simulink model "ACDCMG_sim8"  (R2022a)
settings: Solver=FixedStepAuto  StartTime=0.0  StopTime=0.5  FixedStep=Ts  MaxStep=1e-2  RelTol=1e-3
InitFcn:
  | Set_parameters_R2018
values from neighbouring files (symbols this model uses):
  D_invs = 0.05    [Set_parameters_R2018.m]
  dis11 = 3    [Set_parameters_R2018.m]
  dis12 = 3    [Set_parameters_R2018.m]
  dis2 = 0.2    [Set_parameters_R2018.m]
  dis3 = 0.15    [Set_parameters_R2018.m]
  dis4 = 0.2    [Set_parameters_R2018.m]
  dis5 = 0.25    [Set_parameters_R2018.m]
  dis6 = 0.1    [Set_parameters_R2018.m]
  Fnom = 60    [Set_parameters_R2018.m]
  H_invs = 6    [Set_parameters_R2018.m]
  max_min = 1    [Set_parameters_R2018.m]
  P_Load_3 = S_Load_3* PF_Load_3    (= 7650)    [Set_parameters_R2018.m]
  P_nom_inv = 3e3    (= 3000)    [Set_parameters_R2018.m]
  Pnom_T1 = 1.5e6    (= 1500000)    [Set_parameters_R2018.m]
  Pnom_T2 = 1.5e6    (= 1500000)    [Set_parameters_R2018.m]
  Pnom_T3 = 4e6    (= 4000000)    [Set_parameters_R2018.m]
  Ql_Load_3 = S_Load_3 * sin(acos(PF_Load_3))    [Set_parameters_R2018.m]
  R_Load_9 = (Vnom_prim * 1.35)^2 / P_Load_9    (= 1084.6153125)    [Set_parameters_R2018.m]
  R_Load_DC = Vnom_DC^2/ P_Load_DC    (= 45)    [Set_parameters_R2018.m]
  Rl = 0.17    [Set_parameters_R2018.m]
  Rls = 0.013    [Set_parameters_R2018.m]
  Ts = Ts_Power    (= 6.94444444444e-06)    [Set_parameters_R2018.m]
  Ts_Control = 6*Ts_Power    (= 4.16666666667e-05)    [Set_parameters_R2018.m]
  Ts_Inv = 0.07    [Set_parameters_R2018.m]
  Ts_Power = 1/(24*Fnom)/100    (= 6.94444444444e-06)    [Set_parameters_R2018.m]
  Ts_PV = 0.05    [Set_parameters_R2018.m]
  V1_LL_T3 = 69e3    (= 69000)    [Set_parameters_R2018.m]
  Vmin_mppt = 100    [Set_parameters_R2018.m]
  Vnom_DC = 300    [Set_parameters_R2018.m]
  Vnom_Diesel = 2.4e3    (= 2400)    [Set_parameters_R2018.m]
  Vnom_prim = 13.8e3    (= 13800)    [Set_parameters_R2018.m]
  Vnom_sec = 220    [Set_parameters_R2018.m]
  Vnom_ter_AC_DC = 150    [Set_parameters_R2018.m]
  Xl = 0.3    [Set_parameters_R2018.m]
  Xls = 0.93e-3    (= 0.00093)    [Set_parameters_R2018.m]
undefined symbols (not defined in the file or in its folder): D1, dEgdT, Delta, DiscIntNeverNeededParam, EgRef, fn, gcbh, Ion, k1, Lithium, Rsh_array5pc, sps_rtmsupport, Tref_K, VnInv, VT_ref
libraries: spsCurrentMeasurementLib x40, spsRMSLib x29, spsSeriesRLCBranchLib x23, spsVoltageMeasurementLib x21, spsMeanLib x14, spsThreePhaseVIMeasurementLib x14, powerlib_extras x13, spsThreePhaseSeriesRLCBranchLib x12, spsPower3phInstantaneousLib x10, spsBreakerLib x8, spsControlledVoltageSourceLib x8, spsPowerLib x8
(part 2 of 12)

== system ACDCMG_sim8/SM_Grid_Simulation/Boost converter DC //DC 2 5 kHz - 300V  ==
  note: DC_PV Bus
  note: DC bus Bus
  note: 5 kHz - 300V
      | Boost Converter
  note: 10.5-kW Grid-Connected PV Array (Detailed Model)
  " " : Subsystem  mask(Boost Control - MPPT){fc=5000, T_MPPT=200e-6, Dinit=0.25}
      mask prompts: fc "PWM switching frequency (Hz)"; T_MPPT "Time window used by MPPT control (s)"; Dinit "Initial value of duty cycle"
      mask Display: image('Icons\FPGA.png');
  C1 : spsSeriesRLCBranchLib/Series RLC Branch  LConnTagsString=__new0  RConnTagsString=__new0  BranchType=C  Resistance=1.0  Inductance=1.0  SetiL0=off  InitialCurrent=0  Capacitance=1200e-6  Setx0=off  InitialVoltage=0  Measurements=None
  C3 : spsSeriesRLCBranchLib/Series RLC Branch  LConnTagsString=__new0  RConnTagsString=__new0  BranchType=C  Resistance=1.0  Inductance=1.0  SetiL0=off  InitialCurrent=0  Capacitance=100e-6  Setx0=off  InitialVoltage=0  Measurements=Branch voltage
  Current Measurement1 : spsCurrentMeasurementLib/Current Measurement  PhasorSimulation=off  OutputType=Complex  PSBequivalent=0
  Current Measurement2 : spsCurrentMeasurementLib/Current Measurement  PhasorSimulation=off  OutputType=Complex  PSBequivalent=0
  Diode1 : spsDiodeLib/Diode  Ron=1e-4  Lon=0  Vf=0  IC=0  UseSnubber=off  Rs=inf  Cs=inf  Measurements=off
  Display{2..4,6} (4 alike) : Display
  IGBT1 : spsIGBTLib/IGBT  Ron=0.001  Lon=0  Vf=0  Tf=0  Tt=0  IC=0  Rs=1e5  Cs=inf  Measurements=off
  L1 : spsSeriesRLCBranchLib/Series RLC Branch  LConnTagsString=__new0  RConnTagsString=__new0  BranchType=RL  Resistance=0.005  Inductance=9e-3  SetiL0=off  InitialCurrent=0  Capacitance=1e-6  Setx0=off  InitialVoltage=0  Measurements=None
  Mean : spsMeanLib/Mean  Freq=10  Vinit=0  Ts=0
  Mean1 : spsMeanLib/Mean  Freq=10  Vinit=0  Ts=0
  Product : Product
  Step : Step  Time=0  SampleTime=0
  "Vdc " : spsVoltageMeasurementLib/Voltage Measurement  Tag=PoWeRsYsTeMmEaSuReMeNt  PhasorSimulation=off  OutputType=Magnitude  PSBequivalent=0
  Vdc 1 : spsVoltageMeasurementLib/Voltage Measurement  Tag=PoWeRsYsTeMmEaSuReMeNt  PhasorSimulation=off  OutputType=Magnitude  PSBequivalent=0
  B + : PMIOPort  Side=Right
  + : PMIOPort  Port=2  Side=Left
  - : PMIOPort  Port=3  Side=Left
  B - : PMIOPort  Port=4  Side=Right
  tag scope: I_DC_bus_PV=global, V_DC_bus_PV=global, g_boost_PV=global
  wires:
  [I_PV] -> " "/2(I_PV)
  " "/1(Pulses) -> Product/2
  [V_PV] -> " "/1(V_PV)
  Step/1 -> Product/1
  Current Measurement2/1 -> Mean1/1
  Mean/1 -> Display6/1
  Current Measurement1/1 -> [I_DC_bus_PV], Mean/1
  "Vdc "/1 -> Display3/1, [V_DC_bus_PV]
  Product/1 -> [g_boost_PV]
  [g_boost_PV] -> IGBT1/1
  Vdc 1/1 -> Display4/1
  Mean1/1 -> Display2/1
  connections:
  Current Measurement2/RConn1 -- Vdc 1/LConn1 -- L1/LConn1 -- C3/LConn1
  C3/RConn1 -- -/RConn1 -- C1/RConn1 -- "Vdc "/LConn2 -- IGBT1/RConn1 -- B -/RConn1 -- Vdc 1/LConn2
  IGBT1/LConn1 -- Diode1/LConn1 -- L1/RConn1
  +/RConn1 -- Current Measurement1/RConn1
  C1/LConn1 -- Current Measurement1/LConn1 -- Diode1/RConn1 -- "Vdc "/LConn1
  B +/RConn1 -- Current Measurement2/LConn1

== system ACDCMG_sim8/SM_Grid_Simulation/Bus_1 ==
  Mux : Mux  Inputs=2
  "Power (3ph, Instantaneous)" : spsPower3phInstantaneousLib/Power (3ph, Instantaneous)
  Power Factor Block1 : Subsystem  mask(Power Factor Block){Freq=Fnom, Vinit=[0, 0], Iinit=[0, 0], Ts=0}
      mask prompts: Freq "Fundamental frequency (Hz):"; Vinit "Voltage initial input [ Mag, Phase (degrees) ]:"; Iinit "Current initial input [ Mag, Phase (degrees) ]:"; Ts "Sample time:"
      mask help:
      | Power Factor Block developed by Dr Rodney Tan
      | Version 1.01 (Aug 2016)
      |
      | Compute power factor and phase angle of AC circuit voltage-current pair at fundamental frequency.
      |
      | The computation is based on Power block and Complex number function block.
      |
      | For the first cycle of simulation, the outputs are held constant to the powers computed for the Voltage initial input and Current initial input parameters.
      mask Help:
      | <b>Fundamental Frequency (Hz)</b>
      | Specify the measurement fundamental frequency, in hertz, of the input signal.
      | 
      | <b>Voltage initial input [ Mag, Phase (degrees) ]</b>
      | Specify the voltage initial magnitude and phase to set a constant output for the first cycle of simulation.
      | 
      | <b>Current initial input [ Mag, Phase (degrees) ]</b>
      | Specify the current initial magnitude and phase to set a constant output for the first cycle of simulation.
      | 
      | <b>Sample Time</b>
      | Specify the sample time of the block, in seconds. Set to 0 to implement a continuous block.
      mask TypeOptions Freq: Power/Freq
      mask TypeOptions Vinit: Power/Vinit
      mask TypeOptions Iinit: Power/Iinit
      mask TypeOptions Ts: Power/Ts
  "Means_Bus1      " : Outport  VectorParamsAs1DForOutWhenUnconnected=off
  tag scope: Bus1_Iabc=global, Bus1_P=global, Bus1_Q=global, Bus1_Vabc=global
  wires:
  [IabcLL_Bus_1] -> "Power (3ph, Instantaneous)"/2, Power Factor Block1/2(Iabc), Mux/2  "Iabc"
  Mux/1 -> "Means_Bus1      "/1
  Power Factor Block1/2("Iabc y Iabc ") -> [Bus1_Iabc]
  Power Factor Block1/1("Vabc y Vabc ") -> [Bus1_Vabc]
  [VabcLL_Bus_1] -> Power Factor Block1/1(Vabc), "Power (3ph, Instantaneous)"/1, Mux/1  "Vabc"
  "Power (3ph, Instantaneous)"/1 -> [Bus1_P]
  "Power (3ph, Instantaneous)"/2 -> [Bus1_Q]

== system ACDCMG_sim8/SM_Grid_Simulation/Bus_14 1 ==
  " r1_ L13" : Constant  Value=Rl
  Active powers losses A : Display
      settings: Format=bank
  Active powers losses B : Display
      settings: Format=bank
  Active powers losses c : Display
      settings: Format=bank
  Math Function : Math  Operator=square  SignedPower=on
  Math Function1 : Math  Operator=square  SignedPower=on
  Math Function2 : Math  Operator=square  SignedPower=on
  Mux : Mux  Inputs=3
  Product : Product
  Product1 : Product
  Product2 : Product
  RMS1 : spsRMSLib/RMS  TrueRMS=on  Freq=60  RMSInit=0  Ts=0
  RMS2 : spsRMSLib/RMS  TrueRMS=on  Freq=60  RMSInit=0  Ts=0
  RMS3 : spsRMSLib/RMS  TrueRMS=on  Freq=60  RMSInit=0  Ts=0
  W_to_kW : Gain  Gain=1e-3
  W_to_kW1 : Gain  Gain=1e-3
  W_to_kW2 : Gain  Gain=1e-3
  tag scope: Bus_14_1_LineA_Ploss=global, Bus_14_1_LineB_Ploss=global, Bus_14_1_LineC_Ploss=global, Power_Losse_abc_L1=global
  wires:
  Math Function/1 -> Product/2
  [Ia_L1] -> RMS2/1
  Math Function1/1 -> Product1/2
  [Ib_L1] -> RMS1/1
  Math Function2/1 -> Product2/2
  " r1_ L13"/1 -> Product2/1, Product1/1, Product/1
  [Ic_L1] -> RMS3/1
  Product/1 -> W_to_kW/1
  Product2/1 -> W_to_kW2/1
  Product1/1 -> W_to_kW1/1
  RMS2/1 -> Math Function/1
  RMS1/1 -> Math Function1/1
  RMS3/1 -> Math Function2/1
  W_to_kW/1 -> [Bus_14_1_LineA_Ploss], Mux/1, Active powers losses A/1  "D_Pa_kW"
  W_to_kW1/1 -> [Bus_14_1_LineB_Ploss], Mux/2, Active powers losses B/1  "D_Pb_kW"
  W_to_kW2/1 -> Active powers losses c/1, [Bus_14_1_LineC_Ploss], Mux/3  "D_Pc_kW"
  Mux/1 -> [Power_Losse_abc_L1]

== system ACDCMG_sim8/SM_Grid_Simulation/Bus_14 2 ==
  " r1_ L13" : Constant  Value=Rls
  Active powers losses A : Display
      settings: Format=bank
  Active powers losses B : Display
      settings: Format=bank
  Active powers losses c : Display
      settings: Format=bank
  Math Function : Math  Operator=square  SignedPower=on
  Math Function1 : Math  Operator=square  SignedPower=on
  Math Function2 : Math  Operator=square  SignedPower=on
  Mux : Mux  Inputs=3
  Product : Product
  Product1 : Product
  Product2 : Product
  RMS1 : spsRMSLib/RMS  TrueRMS=on  Freq=60  RMSInit=0  Ts=0
  RMS2 : spsRMSLib/RMS  TrueRMS=on  Freq=60  RMSInit=0  Ts=0
  RMS3 : spsRMSLib/RMS  TrueRMS=on  Freq=60  RMSInit=0  Ts=0
  W_to_kW : Gain  Gain=1e-3
  W_to_kW1 : Gain  Gain=1e-3
  W_to_kW2 : Gain  Gain=1e-3
  tag scope: Bus_14_2_LineA_Ploss=global, Bus_14_2_LineB_Ploss=global, Bus_14_2_LineC_Ploss=global, Power_Losse_abc_L2=global
  wires:
  Math Function/1 -> Product/2
  [Ia_L2] -> RMS2/1
  Math Function1/1 -> Product1/2
  [Ib_L2] -> RMS1/1
  Math Function2/1 -> Product2/2
  " r1_ L13"/1 -> Product2/1, Product1/1, Product/1
  [Ic_L2] -> RMS3/1
  Product/1 -> W_to_kW/1
  Product2/1 -> W_to_kW2/1
  Product1/1 -> W_to_kW1/1
  RMS2/1 -> Math Function/1
  RMS1/1 -> Math Function1/1
  RMS3/1 -> Math Function2/1
  W_to_kW/1 -> [Bus_14_2_LineA_Ploss], Mux/1, Active powers losses A/1  "D_Pa_kW"
  W_to_kW1/1 -> [Bus_14_2_LineB_Ploss], Mux/2, Active powers losses B/1  "D_Pb_kW"
  W_to_kW2/1 -> Active powers losses c/1, [Bus_14_2_LineC_Ploss], Mux/3  "D_Pc_kW"
  Mux/1 -> [Power_Losse_abc_L2]

== system ACDCMG_sim8/SM_Grid_Simulation/Bus_14 3 ==
  " r1_ L13" : Constant  Value=Rl
  Active powers losses A : Display  Commented=on
      settings: Format=bank
  Active powers losses B : Display  Commented=on
      settings: Format=bank
  Active powers losses c : Display  Commented=on
      settings: Format=bank
  "Delta Pabc " : Scope  NumInputPorts=4
  Math Function : Math  Operator=square  SignedPower=on
  Math Function1 : Math  Operator=square  SignedPower=on
  Math Function2 : Math  Operator=square  SignedPower=on
  Mux : Mux  Inputs=3
  Product : Product
  Product1 : Product
  Product2 : Product
  RMS1 : spsRMSLib/RMS  TrueRMS=on  Freq=60  RMSInit=0  Ts=0
  RMS2 : spsRMSLib/RMS  TrueRMS=on  Freq=60  RMSInit=0  Ts=0
  RMS3 : spsRMSLib/RMS  TrueRMS=on  Freq=60  RMSInit=0  Ts=0
  W_to_kW : Gain  Gain=1e-3
  W_to_kW1 : Gain  Gain=1e-3
  W_to_kW2 : Gain  Gain=1e-3
  tag scope: Bus_14_3_LineA_Ploss=global, Bus_14_3_LineB_Ploss=global, Bus_14_3_LineC_Ploss=global, Power_Losse_abc_L3=global
  wires:
  Math Function/1 -> Product/2
  [Ia_L3] -> RMS2/1
  Math Function1/1 -> Product1/2
  [Ib_L3] -> RMS1/1
  Math Function2/1 -> Product2/2
  " r1_ L13"/1 -> Product2/1, Product1/1, Product/1
  [Ic_L3] -> RMS3/1
  Product/1 -> W_to_kW/1
  Product2/1 -> W_to_kW2/1
  Product1/1 -> W_to_kW1/1
  RMS2/1 -> Math Function/1
  RMS1/1 -> Math Function1/1
  RMS3/1 -> Math Function2/1
  W_to_kW/1 -> Mux/1, [Bus_14_3_LineA_Ploss], Active powers losses A/1  "D_Pa_kW"
  W_to_kW1/1 -> Mux/2, [Bus_14_3_LineB_Ploss], Active powers losses B/1  "D_Pb_kW"
  W_to_kW2/1 -> Active powers losses c/1, Mux/3, [Bus_14_3_LineC_Ploss]  "D_Pc_kW"
  Mux/1 -> [Power_Losse_abc_L3]

== system ACDCMG_sim8/SM_Grid_Simulation/Bus_14 4 ==
  " r1_ L13" : Constant  Value=Rls
  Active powers losses A : Display
      settings: Format=bank
  Active powers losses B : Display
      settings: Format=bank
  Active powers losses c : Display
      settings: Format=bank
  Math Function : Math  Operator=square  SignedPower=on
  Math Function1 : Math  Operator=square  SignedPower=on
  Math Function2 : Math  Operator=square  SignedPower=on
  Mux : Mux  Inputs=3
  Product : Product
  Product1 : Product
  Product2 : Product
  RMS1 : spsRMSLib/RMS  TrueRMS=on  Freq=60  RMSInit=0  Ts=0
  RMS2 : spsRMSLib/RMS  TrueRMS=on  Freq=60  RMSInit=0  Ts=0
  RMS3 : spsRMSLib/RMS  TrueRMS=on  Freq=60  RMSInit=0  Ts=0
  W_to_kW : Gain  Gain=1e-3
  W_to_kW1 : Gain  Gain=1e-3
  W_to_kW2 : Gain  Gain=1e-3
  tag scope: Bus_14_4_LineA_Ploss=global, Bus_14_4_LineB_Ploss=global, Bus_14_4_LineC_Ploss=global, Power_Losse_abc_L4=global
  wires:
  Math Function/1 -> Product/2
  [Ia_L4] -> RMS2/1
  Math Function1/1 -> Product1/2
  [Ib_L4] -> RMS1/1
  Math Function2/1 -> Product2/2
  " r1_ L13"/1 -> Product2/1, Product1/1, Product/1
  [Ic_L4] -> RMS3/1
  Product/1 -> W_to_kW/1
  Product2/1 -> W_to_kW2/1
  Product1/1 -> W_to_kW1/1
  RMS2/1 -> Math Function/1
  RMS1/1 -> Math Function1/1
  RMS3/1 -> Math Function2/1
  W_to_kW/1 -> Mux/1, [Bus_14_4_LineA_Ploss], Active powers losses A/1  "D_Pa_kW"
  W_to_kW1/1 -> Mux/2, [Bus_14_4_LineB_Ploss], Active powers losses B/1  "D_Pb_kW"
  W_to_kW2/1 -> Active powers losses c/1, [Bus_14_4_LineC_Ploss], Mux/3  "D_Pc_kW"
  Mux/1 -> [Power_Losse_abc_L4]

== system ACDCMG_sim8/SM_Grid_Simulation/Bus_14 5 ==
  " r1_ L13" : Constant  Value=Rls
  Active powers losses A : Display
      settings: Format=bank
  Active powers losses B : Display
      settings: Format=bank
  Active powers losses c : Display
      settings: Format=bank
  Math Function : Math  Operator=square  SignedPower=on
  Math Function1 : Math  Operator=square  SignedPower=on
  Math Function2 : Math  Operator=square  SignedPower=on
  Mux : Mux  Inputs=3
  Product : Product
  Product1 : Product
  Product2 : Product
  RMS1 : spsRMSLib/RMS  TrueRMS=on  Freq=60  RMSInit=0  Ts=0
  RMS2 : spsRMSLib/RMS  TrueRMS=on  Freq=60  RMSInit=0  Ts=0
  RMS3 : spsRMSLib/RMS  TrueRMS=on  Freq=60  RMSInit=0  Ts=0
  W_to_kW : Gain  Gain=1e-3
  W_to_kW1 : Gain  Gain=1e-3
  W_to_kW2 : Gain  Gain=1e-3
  tag scope: Bus_14_5_LineA_Ploss=global, Bus_14_5_LineB_Ploss=global, Bus_14_5_LineC_Ploss=global, Power_Losse_abc_L5=global
  wires:
  Math Function/1 -> Product/2
  [Ia_L5] -> RMS2/1
  Math Function1/1 -> Product1/2
  [Ib_L5] -> RMS1/1
  Math Function2/1 -> Product2/2
  " r1_ L13"/1 -> Product2/1, Product1/1, Product/1
  [Ic_L5] -> RMS3/1
  Product/1 -> W_to_kW/1
  Product2/1 -> W_to_kW2/1
  Product1/1 -> W_to_kW1/1
  RMS2/1 -> Math Function/1
  RMS1/1 -> Math Function1/1
  RMS3/1 -> Math Function2/1
  W_to_kW/1 -> [Bus_14_5_LineA_Ploss], Mux/1, Active powers losses A/1  "D_Pa_kW"
  W_to_kW1/1 -> [Bus_14_5_LineB_Ploss], Mux/2, Active powers losses B/1  "D_Pb_kW"
  W_to_kW2/1 -> Active powers losses c/1, [Bus_14_5_LineC_Ploss], Mux/3  "D_Pc_kW"
  Mux/1 -> [Power_Losse_abc_L5]

== system ACDCMG_sim8/SM_Grid_Simulation/Bus_14 6 ==
  " r1_ L13" : Constant  Value=Rls
  Active powers losses A : Display
      settings: Format=bank
  Active powers losses B : Display
      settings: Format=bank
  Active powers losses c : Display
      settings: Format=bank
  Math Function : Math  Operator=square  SignedPower=on
  Math Function1 : Math  Operator=square  SignedPower=on
  Math Function2 : Math  Operator=square  SignedPower=on
  Mux : Mux  Inputs=3
  Product : Product
  Product1 : Product
  Product2 : Product
  RMS1 : spsRMSLib/RMS  TrueRMS=on  Freq=60  RMSInit=0  Ts=0
  RMS2 : spsRMSLib/RMS  TrueRMS=on  Freq=60  RMSInit=0  Ts=0
  RMS3 : spsRMSLib/RMS  TrueRMS=on  Freq=60  RMSInit=0  Ts=0
  W_to_kW : Gain  Gain=1e-3
  W_to_kW1 : Gain  Gain=1e-3
  W_to_kW2 : Gain  Gain=1e-3
  tag scope: Bus_14_6_LineA_Ploss=global, Bus_14_6_LineB_Ploss=global, Bus_14_6_LineC_Ploss=global, Power_Losse_abc_L6=global
  wires:
  Math Function/1 -> Product/2
  [Ia_L6] -> RMS2/1
  Math Function1/1 -> Product1/2
  [Ib_L6] -> RMS1/1
  Math Function2/1 -> Product2/2
  " r1_ L13"/1 -> Product2/1, Product1/1, Product/1
  [Ic_L6] -> RMS3/1
  Product/1 -> W_to_kW/1
  Product2/1 -> W_to_kW2/1
  Product1/1 -> W_to_kW1/1
  RMS2/1 -> Math Function/1
  RMS1/1 -> Math Function1/1
  RMS3/1 -> Math Function2/1
  W_to_kW/1 -> [Bus_14_6_LineA_Ploss], Mux/1, Active powers losses A/1  "D_Pa_kW"
  W_to_kW1/1 -> [Bus_14_6_LineB_Ploss], Mux/2, Active powers losses B/1  "D_Pb_kW"
  W_to_kW2/1 -> Active powers losses c/1, [Bus_14_6_LineC_Ploss], Mux/3  "D_Pc_kW"
  Mux/1 -> [Power_Losse_abc_L6]

== system ACDCMG_sim8/SM_Grid_Simulation/Bus_14 7 ==
  " r1_ L13" : Constant  Value=Rls
  Active powers losses A : Display
      settings: Format=bank
  Active powers losses B : Display
      settings: Format=bank
  Active powers losses c : Display
      settings: Format=bank
  Math Function : Math  Operator=square  SignedPower=on
  Math Function1 : Math  Operator=square  SignedPower=on
  Math Function2 : Math  Operator=square  SignedPower=on
  Mux : Mux  Inputs=3
  Product : Product
  Product1 : Product
  Product2 : Product
  RMS1 : spsRMSLib/RMS  TrueRMS=on  Freq=60  RMSInit=0  Ts=0
  RMS2 : spsRMSLib/RMS  TrueRMS=on  Freq=60  RMSInit=0  Ts=0
  RMS3 : spsRMSLib/RMS  TrueRMS=on  Freq=60  RMSInit=0  Ts=0
  W_to_kW : Gain  Gain=1e-3
  W_to_kW1 : Gain  Gain=1e-3
  W_to_kW2 : Gain  Gain=1e-3
  tag scope: Bus_14_7_LineA_Ploss=global, Bus_14_7_LineB_Ploss=global, Bus_14_7_LineC_Ploss=global, Power_Losse_abc_L7=global
  wires:
  Math Function/1 -> Product/2
  [Ia_L7] -> RMS2/1
  Math Function1/1 -> Product1/2
  [Ib_L7] -> RMS1/1
  Math Function2/1 -> Product2/2
  " r1_ L13"/1 -> Product2/1, Product1/1, Product/1
  [Ic_L7] -> RMS3/1
  Product/1 -> W_to_kW/1
  Product2/1 -> W_to_kW2/1
  Product1/1 -> W_to_kW1/1
  RMS2/1 -> Math Function/1
  RMS1/1 -> Math Function1/1
  RMS3/1 -> Math Function2/1
  W_to_kW/1 -> [Bus_14_7_LineA_Ploss], Mux/1, Active powers losses A/1  "D_Pa_kW"
  W_to_kW1/1 -> [Bus_14_7_LineB_Ploss], Mux/2, Active powers losses B/1  "D_Pb_kW"
  W_to_kW2/1 -> Active powers losses c/1, [Bus_14_7_LineC_Ploss], Mux/3  "D_Pc_kW"
  Mux/1 -> [Power_Losse_abc_L7]

== system ACDCMG_sim8/SM_Grid_Simulation/Bus_2 ==
  "Power (3ph, Instantaneous)" : spsPower3phInstantaneousLib/Power (3ph, Instantaneous)
  Power Factor Block1 : Subsystem  mask(Power Factor Block){Freq=Fnom, Vinit=[0, 0], Iinit=[0, 0], Ts=0}
      mask prompts: Freq "Fundamental frequency (Hz):"; Vinit "Voltage initial input [ Mag, Phase (degrees) ]:"; Iinit "Current initial input [ Mag, Phase (degrees) ]:"; Ts "Sample time:"
      mask help:
      | Power Factor Block developed by Dr Rodney Tan
      | Version 1.01 (Aug 2016)
      |
      | Compute power factor and phase angle of AC circuit voltage-current pair at fundamental frequency.
      |
      | The computation is based on Power block and Complex number function block.
      |
      | For the first cycle of simulation, the outputs are held constant to the powers computed for the Voltage initial input and Current initial input parameters.
      mask Help:
      | <b>Fundamental Frequency (Hz)</b>
      | Specify the measurement fundamental frequency, in hertz, of the input signal.
      | 
      | <b>Voltage initial input [ Mag, Phase (degrees) ]</b>
      | Specify the voltage initial magnitude and phase to set a constant output for the first cycle of simulation.
      | 
      | <b>Current initial input [ Mag, Phase (degrees) ]</b>
      | Specify the current initial magnitude and phase to set a constant output for the first cycle of simulation.
      | 
      | <b>Sample Time</b>
      | Specify the sample time of the block, in seconds. Set to 0 to implement a continuous block.
      mask TypeOptions Freq: Power/Freq
      mask TypeOptions Vinit: Power/Vinit
      mask TypeOptions Iinit: Power/Iinit
      mask TypeOptions Ts: Power/Ts
  tag scope: Bus2_Iabc=global, Bus2_P=global, Bus2_Q=global, Bus2_Vabc=global
  wires:
  [IabcLL_Bus_2] -> "Power (3ph, Instantaneous)"/2, Power Factor Block1/2(Iabc)
  [VabcLL_Bus_2] -> "Power (3ph, Instantaneous)"/1, Power Factor Block1/1(Vabc)  "Vabc"
  "Power (3ph, Instantaneous)"/1 -> [Bus2_P]
  "Power (3ph, Instantaneous)"/2 -> [Bus2_Q]
  Power Factor Block1/1("Vabc y Vabc ") -> [Bus2_Vabc]
  Power Factor Block1/2("Iabc y Iabc ") -> [Bus2_Iabc]

== system ACDCMG_sim8/SM_Grid_Simulation/Bus_3 ==
  "Power (3ph, Instantaneous)" : spsPower3phInstantaneousLib/Power (3ph, Instantaneous)
  Power Factor Block1 : Subsystem  mask(Power Factor Block){Freq=Fnom, Vinit=[0, 0], Iinit=[0, 0], Ts=0}
      mask prompts: Freq "Fundamental frequency (Hz):"; Vinit "Voltage initial input [ Mag, Phase (degrees) ]:"; Iinit "Current initial input [ Mag, Phase (degrees) ]:"; Ts "Sample time:"
      mask help:
      | Power Factor Block developed by Dr Rodney Tan
      | Version 1.01 (Aug 2016)
      |
      | Compute power factor and phase angle of AC circuit voltage-current pair at fundamental frequency.
      |
      | The computation is based on Power block and Complex number function block.
      |
      | For the first cycle of simulation, the outputs are held constant to the powers computed for the Voltage initial input and Current initial input parameters.
      mask Help:
      | <b>Fundamental Frequency (Hz)</b>
      | Specify the measurement fundamental frequency, in hertz, of the input signal.
      | 
      | <b>Voltage initial input [ Mag, Phase (degrees) ]</b>
      | Specify the voltage initial magnitude and phase to set a constant output for the first cycle of simulation.
      | 
      | <b>Current initial input [ Mag, Phase (degrees) ]</b>
      | Specify the current initial magnitude and phase to set a constant output for the first cycle of simulation.
      | 
      | <b>Sample Time</b>
      | Specify the sample time of the block, in seconds. Set to 0 to implement a continuous block.
      mask TypeOptions Freq: Power/Freq
      mask TypeOptions Vinit: Power/Vinit
      mask TypeOptions Iinit: Power/Iinit
      mask TypeOptions Ts: Power/Ts
  tag scope: Bus3_Iabc=global, Bus3_P=global, Bus3_Q=global, Bus3_Vabc=global
  wires:
  [IabcLL_Bus_3] -> "Power (3ph, Instantaneous)"/2, Power Factor Block1/2(Iabc)
  [VabcLL_Bus_3] -> "Power (3ph, Instantaneous)"/1, Power Factor Block1/1(Vabc)  "Signal Vabc"
  "Power (3ph, Instantaneous)"/1 -> [Bus3_P]
  "Power (3ph, Instantaneous)"/2 -> [Bus3_Q]
  Power Factor Block1/1(Vabc y Vabc) -> [Bus3_Vabc]
  Power Factor Block1/2("Iabc y Iabc ") -> [Bus3_Iabc]

== system ACDCMG_sim8/SM_Grid_Simulation/Bus_4 ==
  "Power (3ph, Instantaneous)" : spsPower3phInstantaneousLib/Power (3ph, Instantaneous)
  Power Factor Block1 : Subsystem  mask(Power Factor Block){Freq=Fnom, Vinit=[0, 0], Iinit=[0, 0], Ts=0}
      mask prompts: Freq "Fundamental frequency (Hz):"; Vinit "Voltage initial input [ Mag, Phase (degrees) ]:"; Iinit "Current initial input [ Mag, Phase (degrees) ]:"; Ts "Sample time:"
      mask help:
      | Power Factor Block developed by Dr Rodney Tan
      | Version 1.01 (Aug 2016)
      |
      | Compute power factor and phase angle of AC circuit voltage-current pair at fundamental frequency.
      |
      | The computation is based on Power block and Complex number function block.
      |
      | For the first cycle of simulation, the outputs are held constant to the powers computed for the Voltage initial input and Current initial input parameters.
      mask Help:
      | <b>Fundamental Frequency (Hz)</b>
      | Specify the measurement fundamental frequency, in hertz, of the input signal.
      | 
      | <b>Voltage initial input [ Mag, Phase (degrees) ]</b>
      | Specify the voltage initial magnitude and phase to set a constant output for the first cycle of simulation.
      | 
      | <b>Current initial input [ Mag, Phase (degrees) ]</b>
      | Specify the current initial magnitude and phase to set a constant output for the first cycle of simulation.
      | 
      | <b>Sample Time</b>
      | Specify the sample time of the block, in seconds. Set to 0 to implement a continuous block.
      mask TypeOptions Freq: Power/Freq
      mask TypeOptions Vinit: Power/Vinit
      mask TypeOptions Iinit: Power/Iinit
      mask TypeOptions Ts: Power/Ts
  tag scope: Bus4_Iabc=global, Bus4_P=global, Bus4_Q=global, Bus4_Vabc=global
  wires:
  [IabcLL_Bus_4] -> "Power (3ph, Instantaneous)"/2, Power Factor Block1/2(Iabc)
  Power Factor Block1/2("Iabc y Iabc ") -> [Bus4_Iabc]
  Power Factor Block1/1(Vabc y Vabc) -> [Bus4_Vabc]
  [VabcLL_Bus_4] -> "Power (3ph, Instantaneous)"/1, Power Factor Block1/1(Vabc)  "Signal Vabc"
  "Power (3ph, Instantaneous)"/1 -> [Bus4_P]
  "Power (3ph, Instantaneous)"/2 -> [Bus4_Q]

== system ACDCMG_sim8/SM_Grid_Simulation/Bus_5 ==
  "Power (3ph, Instantaneous)" : spsPower3phInstantaneousLib/Power (3ph, Instantaneous)
  Power Factor Block1 : Subsystem  mask(Power Factor Block){Freq=Fnom, Vinit=[0, 0], Iinit=[0, 0], Ts=0}
      mask prompts: Freq "Fundamental frequency (Hz):"; Vinit "Voltage initial input [ Mag, Phase (degrees) ]:"; Iinit "Current initial input [ Mag, Phase (degrees) ]:"; Ts "Sample time:"
      mask help:
      | Power Factor Block developed by Dr Rodney Tan
      | Version 1.01 (Aug 2016)
      |
      | Compute power factor and phase angle of AC circuit voltage-current pair at fundamental frequency.
      |
      | The computation is based on Power block and Complex number function block.
      |
      | For the first cycle of simulation, the outputs are held constant to the powers computed for the Voltage initial input and Current initial input parameters.
      mask Help:
      | <b>Fundamental Frequency (Hz)</b>
      | Specify the measurement fundamental frequency, in hertz, of the input signal.
      | 
      | <b>Voltage initial input [ Mag, Phase (degrees) ]</b>
      | Specify the voltage initial magnitude and phase to set a constant output for the first cycle of simulation.
      | 
      | <b>Current initial input [ Mag, Phase (degrees) ]</b>
      | Specify the current initial magnitude and phase to set a constant output for the first cycle of simulation.
      | 
      | <b>Sample Time</b>
      | Specify the sample time of the block, in seconds. Set to 0 to implement a continuous block.
      mask TypeOptions Freq: Power/Freq
      mask TypeOptions Vinit: Power/Vinit
      mask TypeOptions Iinit: Power/Iinit
      mask TypeOptions Ts: Power/Ts
  tag scope: Bus5_Iabc=global, Bus5_P=global, Bus5_Q=global, Bus5_Vabc=global
  wires:
  [IabcLL_Bus_5] -> Power Factor Block1/2(Iabc), "Power (3ph, Instantaneous)"/2
  Power Factor Block1/2("Iabc y Iabc ") -> [Bus5_Iabc]
  Power Factor Block1/1(Vabc y Vabc) -> [Bus5_Vabc]
  [VabcLL_Bus_5] -> "Power (3ph, Instantaneous)"/1, Power Factor Block1/1(Vabc)  "Signal Vabc"
  "Power (3ph, Instantaneous)"/1 -> [Bus5_P]
  "Power (3ph, Instantaneous)"/2 -> [Bus5_Q]

== system ACDCMG_sim8/SM_Grid_Simulation/Bus_6 ==
  "Power (3ph, Instantaneous)" : spsPower3phInstantaneousLib/Power (3ph, Instantaneous)
  Power Factor Block1 : Subsystem  mask(Power Factor Block){Freq=Fnom, Vinit=[0, 0], Iinit=[0, 0], Ts=0}
      mask prompts: Freq "Fundamental frequency (Hz):"; Vinit "Voltage initial input [ Mag, Phase (degrees) ]:"; Iinit "Current initial input [ Mag, Phase (degrees) ]:"; Ts "Sample time:"
      mask help:
      | Power Factor Block developed by Dr Rodney Tan
      | Version 1.01 (Aug 2016)
      |
      | Compute power factor and phase angle of AC circuit voltage-current pair at fundamental frequency.
      |
      | The computation is based on Power block and Complex number function block.
      |
      | For the first cycle of simulation, the outputs are held constant to the powers computed for the Voltage initial input and Current initial input parameters.
      mask Help:
      | <b>Fundamental Frequency (Hz)</b>
      | Specify the measurement fundamental frequency, in hertz, of the input signal.
      | 
      | <b>Voltage initial input [ Mag, Phase (degrees) ]</b>
      | Specify the voltage initial magnitude and phase to set a constant output for the first cycle of simulation.
      | 
      | <b>Current initial input [ Mag, Phase (degrees) ]</b>
      | Specify the current initial magnitude and phase to set a constant output for the first cycle of simulation.
      | 
      | <b>Sample Time</b>
      | Specify the sample time of the block, in seconds. Set to 0 to implement a continuous block.
      mask TypeOptions Freq: Power/Freq
      mask TypeOptions Vinit: Power/Vinit
      mask TypeOptions Iinit: Power/Iinit
      mask TypeOptions Ts: Power/Ts
  tag scope: Bus6_Iabc=global, Bus6_P=global, Bus6_Q=global, Bus6_Vabc=global
  wires:
  [IabcLL_Bus_6] -> Power Factor Block1/2(Iabc), "Power (3ph, Instantaneous)"/2
  Power Factor Block1/1("Vabc y Vabc ") -> [Bus6_Vabc]
  Power Factor Block1/2(Iabc y Iabc) -> [Bus6_Iabc]
  [VabcLL_Bus_6] -> "Power (3ph, Instantaneous)"/1, Power Factor Block1/1(Vabc)  "Vabc"
  "Power (3ph, Instantaneous)"/1 -> [Bus6_P]
  "Power (3ph, Instantaneous)"/2 -> [Bus6_Q]

== system ACDCMG_sim8/SM_Grid_Simulation/Bus_7 ==
  "Power (3ph, Instantaneous)" : spsPower3phInstantaneousLib/Power (3ph, Instantaneous)
  Power Factor Block1 : Subsystem  mask(Power Factor Block){Freq=Fnom, Vinit=[0, 0], Iinit=[0, 0], Ts=0}
      mask prompts: Freq "Fundamental frequency (Hz):"; Vinit "Voltage initial input [ Mag, Phase (degrees) ]:"; Iinit "Current initial input [ Mag, Phase (degrees) ]:"; Ts "Sample time:"
      mask help:
      | Power Factor Block developed by Dr Rodney Tan
      | Version 1.01 (Aug 2016)
      |
      | Compute power factor and phase angle of AC circuit voltage-current pair at fundamental frequency.
      |
      | The computation is based on Power block and Complex number function block.
      |
      | For the first cycle of simulation, the outputs are held constant to the powers computed for the Voltage initial input and Current initial input parameters.
      mask Help:
      | <b>Fundamental Frequency (Hz)</b>
      | Specify the measurement fundamental frequency, in hertz, of the input signal.
      | 
      | <b>Voltage initial input [ Mag, Phase (degrees) ]</b>
      | Specify the voltage initial magnitude and phase to set a constant output for the first cycle of simulation.
      | 
      | <b>Current initial input [ Mag, Phase (degrees) ]</b>
      | Specify the current initial magnitude and phase to set a constant output for the first cycle of simulation.
      | 
      | <b>Sample Time</b>
      | Specify the sample time of the block, in seconds. Set to 0 to implement a continuous block.
      mask TypeOptions Freq: Power/Freq
      mask TypeOptions Vinit: Power/Vinit
      mask TypeOptions Iinit: Power/Iinit
      mask TypeOptions Ts: Power/Ts
  tag scope: Bus7_Iabc=global, Bus7_P=global, Bus7_Q=global, Bus7_Vabc=global
  wires:
  [IabcLL_Bus_7] -> "Power (3ph, Instantaneous)"/2, Power Factor Block1/2(Iabc)
  [VabcLL_Bus_7] -> "Power (3ph, Instantaneous)"/1, Power Factor Block1/1(Vabc)  "Signal Vabc"
  Power Factor Block1/1(Vabc y Vabc) -> [Bus7_Vabc]
  Power Factor Block1/2("Iabc y Iabc ") -> [Bus7_Iabc]
  "Power (3ph, Instantaneous)"/2 -> [Bus7_Q]
  "Power (3ph, Instantaneous)"/1 -> [Bus7_P]

== system ACDCMG_sim8/SM_Grid_Simulation/Bus_8 ==
  Gain2 : Gain  Commented=on  Gain=Fnom
  Goto2 : Goto  Commented=on  GotoTag=w_iv  TagVisibility=global
  "PMU (PLL-Based, Positive-Sequence)" : spsPMUPLLBasedPositiveSequenceLib/PMU (PLL-Based, Positive-Sequence)  Commented=on  nominalFrequency=60  samplingRate=24  reportingFactor=1
      settings: SourceProductBaseCode=PS
  "Power (3ph, Instantaneous)" : spsPower3phInstantaneousLib/Power (3ph, Instantaneous)
  Power Factor Block1 : Subsystem  mask(Power Factor Block){Freq=Fnom, Vinit=[0, 0], Iinit=[0, 0], Ts=0}
      mask prompts: Freq "Fundamental frequency (Hz):"; Vinit "Voltage initial input [ Mag, Phase (degrees) ]:"; Iinit "Current initial input [ Mag, Phase (degrees) ]:"; Ts "Sample time:"
      mask help:
      | Power Factor Block developed by Dr Rodney Tan
      | Version 1.01 (Aug 2016)
      |
      | Compute power factor and phase angle of AC circuit voltage-current pair at fundamental frequency.
      |
      | The computation is based on Power block and Complex number function block.
      |
      | For the first cycle of simulation, the outputs are held constant to the powers computed for the Voltage initial input and Current initial input parameters.
      mask Help:
      | <b>Fundamental Frequency (Hz)</b>
      | Specify the measurement fundamental frequency, in hertz, of the input signal.
      | 
      | <b>Voltage initial input [ Mag, Phase (degrees) ]</b>
      | Specify the voltage initial magnitude and phase to set a constant output for the first cycle of simulation.
      | 
      | <b>Current initial input [ Mag, Phase (degrees) ]</b>
      | Specify the current initial magnitude and phase to set a constant output for the first cycle of simulation.
      | 
      | <b>Sample Time</b>
      | Specify the sample time of the block, in seconds. Set to 0 to implement a continuous block.
      mask TypeOptions Freq: Power/Freq
      mask TypeOptions Vinit: Power/Vinit
      mask TypeOptions Iinit: Power/Iinit
      mask TypeOptions Ts: Power/Ts
  Scope4 : Scope  Commented=on  NumInputPorts=3
  "Sinusoidal Measurement (PLL, Three-Phase)1" : eeSinusoidalMeasurementV2/Sinusoidal Measurement (PLL, Three-Phase)  Commented=on  Kp_LF=Kp_pll  Ki_LF=Ki_pll  F0=60  Theta0=0  Ts=Ts
      settings: SourceProductBaseCode=PS
  tag scope: Bus8_Iabc=global, Bus8_P=global, Bus8_Q=global, Bus8_Vabc=global
  wires:
  [IabcLL_Bus_8] -> "Power (3ph, Instantaneous)"/2, Power Factor Block1/2(Iabc)
  [VabcLL_Bus_8] -> "Power (3ph, Instantaneous)"/1, Power Factor Block1/1(Vabc)  "Vabc"
  "PMU (PLL-Based, Positive-Sequence)"/3 -> Scope4/3
  "PMU (PLL-Based, Positive-Sequence)"/1 -> Gain2/1, Scope4/1
  Gain2/1 -> Goto2/1
  "PMU (PLL-Based, Positive-Sequence)"/2 -> Scope4/2
  "Power (3ph, Instantaneous)"/1 -> [Bus8_P]
  "Power (3ph, Instantaneous)"/2 -> [Bus8_Q]
  Power Factor Block1/1("Vabc y Vabc ") -> [Bus8_Vabc]
  Power Factor Block1/2("Iabc y Iabc ") -> [Bus8_Iabc]

== system ACDCMG_sim8/SM_Grid_Simulation/Bus_AC//DC3 ==
  note: BUS
  Add : Sum
  Battery system : Subsystem
      mask Display: disp('Open this block\nto display additional \nscopes & measurements')
  Conv pu1 : Gain  Gain=1 /Vnom_DC  SaturateOnIntegerOverflow=on  OutDataTypeStr=Inherit: Same as input  ParamDataTypeStr=Inherit: Same as input
  Display6 : Display
  Gain : Gain  Gain=1/1000
  Mean : spsMeanLib/Mean  Freq=100  Vinit=0  Ts=0
  Mux : Mux  Inputs=1
  PV system : Subsystem
      mask Display: disp('Open this block\nto display additional \nscopes & measurements')
  Product : Product
  tag scope: DC_Bus_Power_kw=global, IDC_Bus=global, P_BusDC=global, V_pu_BusDC=global
  wires:
  Conv pu1/1 -> [VDC_Bus_pu], [V_pu_BusDC]  "DC Voltage (pu)"
  [V_DC_bus] -> Product/1, Conv pu1/1
  Mean/1 -> Mux/1, Product/2, Display6/1
  Product/1 -> Gain/1
  Mux/1 -> [IDC_Bus]
  Gain/1 -> [DC_Bus_Power_kw], [P_BusDC]  "Power (kW)"
  [I_DC_bus_BESS] -> Add/1
  [I_DC_bus_PV] -> Add/2
  Add/1 -> Mean/1

== system ACDCMG_sim8/SM_Grid_Simulation/DATA  ADQUISITION ==
  note: Transformer (T1)
  Power_Losses_abc : Subsystem
  VoltageLL_pu_abc : Subsystem
  scope 11 : Scope
  scope 12 : Scope
  wires:
  [Vabc_Sec_pu] -> scope 11/1
  [Vabc_Prim_pu] -> scope 12/1

== system ACDCMG_sim8/SM_Grid_Simulation/Diesel_ 50MVA ==
  note: Diesel generator 2
  2.4kV  50MVA : spsThreePhaseSeriesRLCBranchLib/Three-Phase Series RLC Branch  LConnTagsString=A|B|C  RConnTagsString=A|B|C  BranchType=RL  Resistance=2.4e3^2/50e6/10  Inductance=2.4e3^2/50e6/(2*pi*60)  Capacitance=1.0  Measurements=None
  Ground1 : spsGroundLib/Ground  LConnTagsString=a
  Programmable Voltage Source1 : spsThreePhaseProgrammableVoltageSourceLib/Three-Phase Programmable Voltage Source  PositiveSequence="[Vnom_Diesel*0.9848 -60  Fnom]"  VariationEntity=None  VariationType=Table of time-amplitude pairs  VariationTypeAlt=Step  VariationStep=-0.3  VariationRate=0.5  VariationMagnitude=0.4  VariationFrequency=2  VariationTiming=[0.1 1.2]  VariationPhaseA=off  Amplitudes=[1]  TimeValues=[0]  HarmonicGeneration=off  HarmonicA=[3 0.2 -25 0]  HarmonicB="[2 0.15  35 2]"  Timing="[0.1  0.6]"  BusType=PV  Pref=Pgen_Diesel  Qref=0  Qmin=-inf  Qmax=inf
  a1 : PMIOPort  Tag=PMCPort  Side=Left
  b1 : PMIOPort  Tag=PMCPort  Port=2  Side=Left
  c1 : PMIOPort  Tag=PMCPort  Port=3  Side=Left
  connections:
  Programmable Voltage Source1/RConn3 -- 2.4kV  50MVA/LConn3
  Ground1/LConn1 -- Programmable Voltage Source1/LConn1
  Programmable Voltage Source1/RConn2 -- 2.4kV  50MVA/LConn2
  2.4kV  50MVA/LConn1 -- Programmable Voltage Source1/RConn1
  b1/RConn1 -- 2.4kV  50MVA/RConn2
  a1/RConn1 -- 2.4kV  50MVA/RConn1
  c1/RConn1 -- 2.4kV  50MVA/RConn3

== system ACDCMG_sim8/SM_Grid_Simulation/Grid Bi-directional Converter 1.1 300 (DC) // 150 V (AC) P_nom 3kW2 ==
  note: Bus DC
  note: Bus AC
  note: Inverter mode:
      |
      | m = 1.2
      | alpha = 0
      |
      | P = 1 kW x 3 phase
      | Q = 1 kVAr x3 phase
      | PF = 0.6
      | Vpu = 0.95
  note: Operation modes
  note: Rectif mode:
      |
      | m = 1
      | alpha = 228
      |
      | P = 975 kVA (DC)
  Means : Inport
  C1 : spsSeriesRLCBranchLib/Series RLC Branch  LConnTagsString=__new0  RConnTagsString=__new0  BranchType=C  Resistance=22.5  Inductance=1e-3  SetiL0=off  InitialCurrent=0  Capacitance=1200e-6  Setx0=off  InitialVoltage=150  Measurements=None
  Control of Inverter : Subsystem
      mask Display: image('Icons\FPGA.png');
  Ground1 : spsGroundLib/Ground  LConnTagsString=a
  Scope : Scope
  Three-Phase Parallel RLC Branch1 : spsThreePhaseParallelRLCBranchLib/Three-Phase Parallel RLC Branch  LConnTagsString=A|B|C  RConnTagsString=A|B|C  BranchType=C  Resistance=1  Inductance=1e-3  Capacitance=2.65e-6  Measurements=None
      settings: SourceProductBaseCode=PS
  Three-Phase Series RLC Branch1 : spsThreePhaseSeriesRLCBranchLib/Three-Phase Series RLC Branch  LConnTagsString=A|B|C  RConnTagsString=A|B|C  BranchType=RL  Resistance=2  Inductance=1e-2  Capacitance=15.5e-5  Measurements=None
  Universal Bridge1 : spsUniversalBridgeLib/Universal Bridge  Arms=3  SnubberResistance=1e5  SnubberCapacitance=inf  Device=MOSFET / Diodes  Ron=1e-3  Lon=0  ForwardVoltages="[  0  0  ]"  ForwardVoltage=0  GTOparameters=[ 10e-6 , 20e-6 ]  IGBTparameters=[ 1e-6 , 2e-6 ]  Measurements=None  Measurements_2=None  converterType=Rectifier
  "a " : PMIOPort  Tag=PMCPort  Side=Left
  b : PMIOPort  Tag=PMCPort  Port=2  Side=Left
  c : PMIOPort  Tag=PMCPort  Port=3  Side=Left
  B1 + : PMIOPort  Port=4  Side=Right
  B1 - : PMIOPort  Port=5  Side=Right
  tag scope: Pulse=global
  wires:
  Control of Inverter/1(Pulses) -> Scope/1, [Pulse]
  [Pulse] -> Universal Bridge1/1
  Means/1 -> Control of Inverter/1(Means)
  connections:
  Three-Phase Series RLC Branch1/RConn1 -- Three-Phase Parallel RLC Branch1/LConn1 -- "a "/RConn1
  Three-Phase Parallel RLC Branch1/LConn2 -- Three-Phase Series RLC Branch1/RConn2 -- b/RConn1
  Three-Phase Parallel RLC Branch1/LConn3 -- Three-Phase Series RLC Branch1/RConn3 -- c/RConn1
  Ground1/LConn1 -- Three-Phase Parallel RLC Branch1/RConn3 -- Three-Phase Parallel RLC Branch1/RConn1 -- Three-Phase Parallel RLC Branch1/RConn2
  Universal Bridge1/LConn3 -- Three-Phase Series RLC Branch1/LConn3
  Three-Phase Series RLC Branch1/LConn2 -- Universal Bridge1/LConn2
  Universal Bridge1/LConn1 -- Three-Phase Series RLC Branch1/LConn1
  B1 +/RConn1 -- C1/LConn1 -- Universal Bridge1/RConn1
  B1 -/RConn1 -- C1/RConn1 -- Universal Bridge1/RConn2

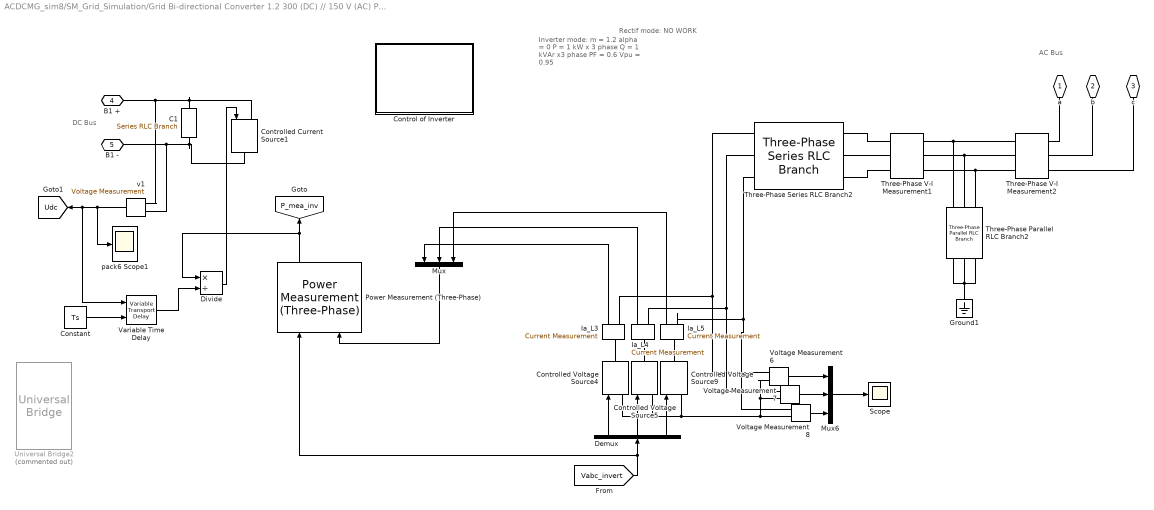
== system ACDCMG_sim8/SM_Grid_Simulation/Grid Bi-directional Converter 1.2 300 (DC) // 150 V (AC) P_nom 3kW3 ==
  note: DC Bus
  note: AC Bus
  note: Inverter mode:
      |
      | m = 1.2
      | alpha = 0
      |
      | P = 1 kW x 3 phase
      | Q = 1 kVAr x3 phase
      | PF = 0.6
      | Vpu = 0.95
  note: Rectif mode:
      |
      | NO WORK
  C1 : spsSeriesRLCBranchLib/Series RLC Branch  LConnTagsString=__new0  RConnTagsString=__new0  BranchType=C  Resistance=22.5  Inductance=1e-3  SetiL0=off  InitialCurrent=0  Capacitance=1200e-6  Setx0=on  InitialVoltage=300  Measurements=None
  Constant : Constant  Value=Ts
  Control of Inverter : Subsystem
      mask Display: image('Icons\FPGA.png');
  Controlled Current Source1 : spsControlledCurrentSourceLib/Controlled Current Source  Initialize=on  Source_Type=AC  Amplitude=0  Phase=0  Frequency=0  Measurements=None
  Controlled Voltage Source4 : spsControlledVoltageSourceLib/Controlled Voltage Source  Initialize=off  Source_Type=AC  Amplitude=VnInv*sqrt(2)  Phase=0  Frequency=fn  Measurements=None
  Controlled Voltage Source5 : spsControlledVoltageSourceLib/Controlled Voltage Source  Initialize=off  Source_Type=AC  Amplitude=VnInv*sqrt(2)  Phase=0  Frequency=fn  Measurements=None
  Controlled Voltage Source9 : spsControlledVoltageSourceLib/Controlled Voltage Source  Initialize=off  Source_Type=AC  Amplitude=VnInv*sqrt(2)  Phase=0  Frequency=fn  Measurements=None
  Demux : Demux  Outputs=3
  Divide : Product  Inputs=*/
  Ground1 : spsGroundLib/Ground  LConnTagsString=a
  Ia_L3 : spsCurrentMeasurementLib/Current Measurement  PhasorSimulation=off  OutputType=Complex  PSBequivalent=0
  Ia_L4 : spsCurrentMeasurementLib/Current Measurement  PhasorSimulation=off  OutputType=Complex  PSBequivalent=0
  Ia_L5 : spsCurrentMeasurementLib/Current Measurement  PhasorSimulation=off  OutputType=Complex  PSBequivalent=0
  Mux : Mux  Inputs=3
  Mux6 : Mux  Inputs=3
  Power Measurement (Three-Phase) : eePowerMeasurement/Power Measurement (Three-Phase)  LabelModeActiveChoice=Continuous  F=60  K=1  Seq=Positive  Ts=0
      settings: SourceProductBaseCode=PS
  Scope : Scope
  Three-Phase Parallel RLC Branch2 : spsThreePhaseParallelRLCBranchLib/Three-Phase Parallel RLC Branch  LConnTagsString=A|B|C  RConnTagsString=A|B|C  BranchType=C  Resistance=1  Inductance=1e-3  Capacitance=2.65e-6  Measurements=None
      settings: SourceProductBaseCode=PS
  Three-Phase Series RLC Branch2 : spsThreePhaseSeriesRLCBranchLib/Three-Phase Series RLC Branch  LConnTagsString=A|B|C  RConnTagsString=A|B|C  BranchType=RL  Resistance=2  Inductance=1e-2  Capacitance=15.5e-5  Measurements=None
  Three-Phase V-I Measurement1 : spsThreePhaseVIMeasurementLib/Three-Phase V-I Measurement  VoltageMeasurement=phase-to-ground  SetLabelV=on  LabelV=u  Vpu=off  VpuLL=off  CurrentMeasurement=yes  SetLabelI=on  LabelI=i  Ipu=off  Pbase=100e6  Vbase=500e3  OutputType=Complex  PhasorSimulation=off  PSBequivalent=0
  Three-Phase V-I Measurement2 : spsThreePhaseVIMeasurementLib/Three-Phase V-I Measurement  VoltageMeasurement=phase-to-ground  SetLabelV=on  LabelV=e  Vpu=off  VpuLL=off  CurrentMeasurement=yes  SetLabelI=on  LabelI=io  Ipu=off  Pbase=100e6  Vbase=500e3  OutputType=Complex  PhasorSimulation=off  PSBequivalent=0
  Universal Bridge2 : spsUniversalBridgeLib/Universal Bridge  Commented=on  Arms=3  SnubberResistance=1e5  SnubberCapacitance=inf  Device=MOSFET / Diodes  Ron=1e-3  Lon=0  ForwardVoltages="[  0  0  ]"  ForwardVoltage=0  GTOparameters=[ 10e-6 , 20e-6 ]  IGBTparameters=[ 1e-6 , 2e-6 ]  Measurements=None  Measurements_2=None  converterType=Rectifier
  Variable Time Delay : VariableTransportDelay  MaximumDelay=2*Ts  InitialOutput=Ts
  Voltage Measurement6 : spsVoltageMeasurementLib/Voltage Measurement  PhasorSimulation=off  OutputType=Complex  PSBequivalent=0
  Voltage Measurement7 : spsVoltageMeasurementLib/Voltage Measurement  PhasorSimulation=off  OutputType=Complex  PSBequivalent=0
  Voltage Measurement8 : spsVoltageMeasurementLib/Voltage Measurement  PhasorSimulation=off  OutputType=Complex  PSBequivalent=0
  pack6 Scope1 : Scope
  v1 : spsVoltageMeasurementLib/Voltage Measurement  PhasorSimulation=off  OutputType=Complex  PSBequivalent=0
  "a " : PMIOPort  Tag=PMCPort  Side=Left
  b : PMIOPort  Tag=PMCPort  Port=2  Side=Left
  c : PMIOPort  Tag=PMCPort  Port=3  Side=Left
  B1 + : PMIOPort  Port=4  Side=Right
  B1 - : PMIOPort  Port=5  Side=Right
  tag scope: P_mea_inv=global, Udc=global
  wires:
  Voltage Measurement8/1 -> Mux6/3
  Mux6/1 -> Scope/1
  Voltage Measurement7/1 -> Mux6/2
  Voltage Measurement6/1 -> Mux6/1
  Demux/3 -> Controlled Voltage Source9/1
  Demux/2 -> Controlled Voltage Source5/1
  Demux/1 -> Controlled Voltage Source4/1
  Ia_L3/1 -> Mux/1
  Ia_L4/1 -> Mux/2
  Ia_L5/1 -> Mux/3
  Mux/1 -> Power Measurement (Three-Phase)/2
  Power Measurement (Three-Phase)/1 -> Divide/1, [P_mea_inv]
  Divide/1 -> Controlled Current Source1/1
  [Vabc_invert] -> Demux/1, Power Measurement (Three-Phase)/1
  Constant/1 -> Variable Time Delay/2
  v1/1 -> pack6 Scope1/1, Variable Time Delay/1, [Udc]
  Variable Time Delay/1 -> Divide/2
  connections:
  Three-Phase V-I Measurement1/RConn1 -- Three-Phase Parallel RLC Branch2/LConn1 -- Three-Phase V-I Measurement2/LConn1
  Three-Phase Parallel RLC Branch2/LConn2 -- Three-Phase V-I Measurement2/LConn2 -- Three-Phase V-I Measurement1/RConn2
  Three-Phase V-I Measurement1/RConn3 -- Three-Phase Parallel RLC Branch2/LConn3 -- Three-Phase V-I Measurement2/LConn3
  Ground1/LConn1 -- Three-Phase Parallel RLC Branch2/RConn3 -- Three-Phase Parallel RLC Branch2/RConn1 -- Three-Phase Parallel RLC Branch2/RConn2
  Ia_L3/RConn1 -- Voltage Measurement6/LConn1 -- Three-Phase Series RLC Branch2/LConn1
  C1/LConn1 -- B1 +/RConn1 -- v1/LConn1 -- Controlled Current Source1/LConn1
  C1/RConn1 -- B1 -/RConn1 -- v1/LConn2 -- Controlled Current Source1/RConn1
  Three-Phase V-I Measurement1/LConn1 -- Three-Phase Series RLC Branch2/RConn1
  Three-Phase V-I Measurement1/LConn2 -- Three-Phase Series RLC Branch2/RConn2
  Three-Phase V-I Measurement1/LConn3 -- Three-Phase Series RLC Branch2/RConn3
  Three-Phase V-I Measurement2/RConn1 -- "a "/RConn1
  Three-Phase V-I Measurement2/RConn2 -- b/RConn1
  Three-Phase V-I Measurement2/RConn3 -- c/RConn1
  Controlled Voltage Source4/LConn1 -- Controlled Voltage Source5/LConn1 -- Controlled Voltage Source9/LConn1 -- Voltage Measurement6/LConn2 -- Voltage Measurement7/LConn2 -- Voltage Measurement8/LConn2
  Ia_L5/RConn1 -- Three-Phase Series RLC Branch2/LConn3 -- Voltage Measurement8/LConn1
  Three-Phase Series RLC Branch2/LConn2 -- Ia_L4/RConn1 -- Voltage Measurement7/LConn1
  Ia_L3/LConn1 -- Controlled Voltage Source4/RConn1
  Ia_L4/LConn1 -- Controlled Voltage Source5/RConn1
  Ia_L5/LConn1 -- Controlled Voltage Source9/RConn1
